simulink model "sampleModel149"  (R2021b)
settings: Solver=VariableStepAuto  StartTime=0.0  StopTime=10.0  RelTol=1e-3
undefined symbols (not defined in the file or in its folder): DiscIntNeverNeededParam, Newton, Raphson
libraries: simulink x9, slpidlib x3
settings Model: Creator=user  LastModifiedBy=user

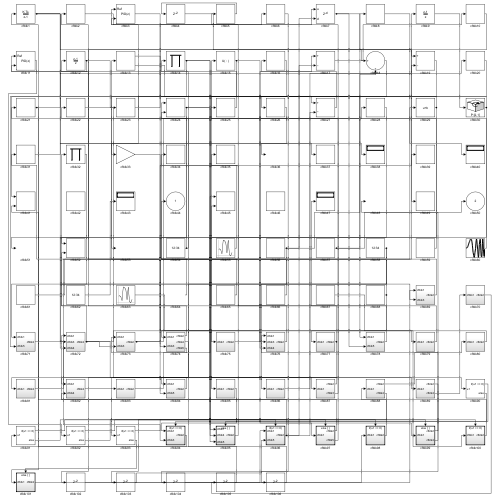
[thumbnail: Simulink's stored preview of the top-level diagram]
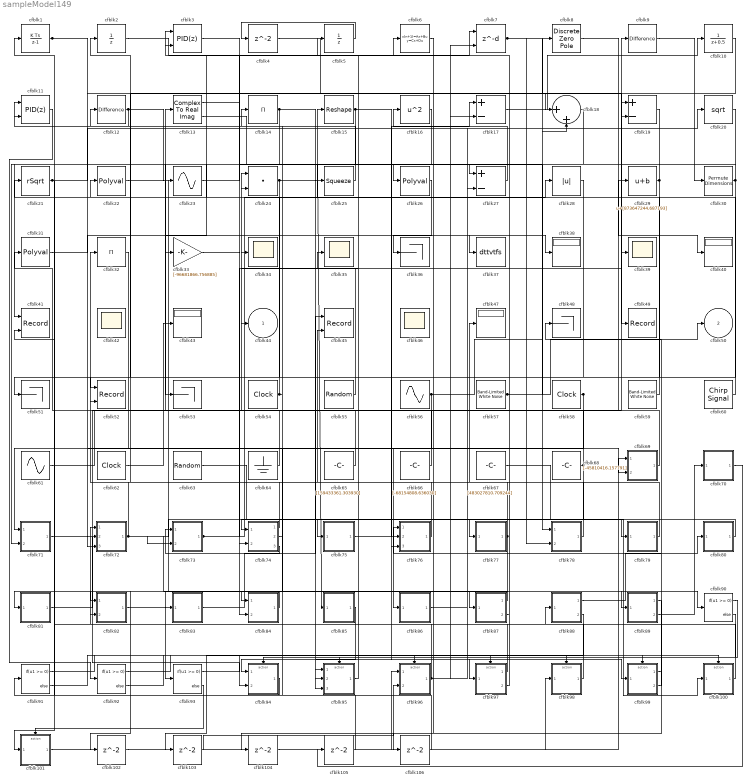
== system sampleModel149 ==
  cfblk1 : DiscreteIntegrator  ICPrevOutput=DiscIntNeverNeededParam  ICPrevScaledInput=DiscIntNeverNeededParam
  cfblk10 : DiscreteTransferFcn  SampleTime=1
  cfblk100 : Subsystem  TreatAsAtomicUnit=on
  cfblk101 : Subsystem  TreatAsAtomicUnit=on
  cfblk{4,102..106} (6 alike) : Delay  SampleTime=1
  cfblk11 : slpidlib/PID Controller (2DOF)  Controller=PID  Form=Parallel  TimeDomain=Discrete-time  UseExternalTs=off  SampleTime=1  IntegratorMethod=Forward Euler  FilterMethod=Forward Euler  ControllerParametersSource=internal  P=1  I=1  D=0  UseFilter=on  N=100  b=1  c=1  TunerSelectOption=Transfer Function Based (PID Tuner App)  InitialConditionSource=internal  InitialConditionForIntegrator=0  InitialConditionForFilter=0  DifferentiatorICPrevScaledInput=0  ExternalReset=none  TrackingMode=off  Kt=1  LimitOutput=off  SatLimitsSource=internal  UpperSaturationLimit=inf  LowerSaturationLimit=-inf  LinearizeAsGain=off  AntiWindupMode=none  Kb=1  POutMin=[]  POutMax=[]  IOutMin=[]  IOutMax=[]  DOutMin=[]  DOutMax=[]  NOutMin=[]  NOutMax=[]  bOutMin=[]  bOutMax=[]  cOutMin=[]  cOutMax=[]  SumOutMin=[]  SumOutMax=[]  SaturationOutMin=[]  SaturationOutMax=[]  PParamMin=[]  PParamMax=[]  IParamMin=[]  IParamMax=[]  DParamMin=[]  DParamMax=[]  NParamMin=[]  NParamMax=[]  bParamMin=[]  bParamMax=[]  cParamMin=[]  cParamMax=[]  KbParamMin=[]  KbParamMax=[]  KtParamMin=[]  KtParamMax=[]  KbOutMin=[]  KbOutMax=[]  KtOutMin=[]  KtOutMax=[]  IntegratorOutMin=[]  IntegratorOutMax=[]  FilterOutMin=[]  FilterOutMax=[]  SumI1OutMin=[]  SumI1OutMax=[]  SumI2OutMin=[]  SumI2OutMax=[]  SumI3OutMin=[]  SumI3OutMax=[]  SumI4OutMin=[]  SumI4OutMax=[]  SumDOutMin=[]  SumDOutMax=[]  Sum1OutMin=[]  Sum1OutMax=[]  Sum2OutMin=[]  Sum2OutMax=[]  Sum3OutMin=[]  Sum3OutMax=[]  DifferentiatorOutMin=[]  DifferentiatorOutMax=[]  FilterDiffOutCoefMin=[]  FilterDiffOutCoefMax=[]  ReciprocalOutMin=[]  ReciprocalOutMax=[]  SumDenOutMin=[]  SumDenOutMax=[]  SumNumOutMin=[]  SumNumOutMax=[]  DivideOutMin=[]  DivideOutMax=[]  UdiffTsProdOutMin=[]  UdiffTsProdOutMax=[]  NTsProdOutMin=[]  NTsProdOutMax=[]  UintegralTsProdOutMin=[]  UintegralTsProdOutMax=[]  UngainTsProdOutMin=[]  UngainTsProdOutMax=[]  IntegratorContinuousStateAttributes=''  IntegratorStateMustResolveToSignalObject=off  IntegratorRTWStateStorageClass=Auto  FilterContinuousStateAttributes=''  FilterStateMustResolveToSignalObject=off  FilterRTWStateStorageClass=Auto  ParallelPVariant=InternalParameters  IdealPVariant=Disabled  IVariant=InternalParameters  DVariant=InternalParameters  bVariant=InternalParameters  cVariant=InternalParameters  IntegratorVariant=Discrete  SatVariant=Disabled  AWVariant=Passthrough  PCopyVariant=Disabled  TRVariant=Disabled  FdbkBlocksVariant=Forward  IdealPFdbkVariant=Disabled  SatFdbkVariant=Disabled  DerivativeFilterVariant=ForwardEulerFilter  NVariant=InternalParameters  NCopyVariant=Disabled  FilterICVariant=InternalICsFilter  IntegratorICVariant=InternalICs  ExternalResetVariant=Disabled  TRSumVariant=Passthrough  SumFdbkVariant=Disabled  SumVariant=Sum_PID  TsampFilterVariant=InternalTs  TsampNgainVariant=Passthrough  TsampIntegralVariant=Passthrough  ExternalSaturationOutDataTypeStr=Inherit: Same as second input
      settings: SourceProductBaseCode=SL
  cfblk12 : simulink/Discrete/Difference  ICPrevInput=0.0  OutMin=[]  OutMax=[]  OutDataTypeStr=Inherit: Inherit via back propagation  OutDataType=fixdt(1, 16)  OutScaling=2^-10  DoSatur=off
  cfblk13 : ComplexToRealImag
  cfblk14 : Product  Inputs=*
  cfblk15 : Reshape
  cfblk16 : Math  Operator=square  SaturateOnIntegerOverflow=on
  cfblk17 : Sum  Inputs=+-
  cfblk18 : Sum  Inputs=|++
  cfblk19 : Sum  Inputs=+-
  cfblk2 : UnitDelay  HasFrameUpgradeWarning=on
  cfblk20 : Sqrt  SaturateOnIntegerOverflow=on
  cfblk21 : Sqrt  Operator=rSqrt  AlgorithmType=Newton-Raphson  SaturateOnIntegerOverflow=on
  cfblk22 : Polyval  Coefs=[ +2.081618890e-019, -1.441693666e-014, +4.719686976e-010, -8.536869453e-006, +1.621573104e-001, -8.087801117e+001 ]
  cfblk23 : Sin  TimeSource=Use external signal  SampleTime=0
  cfblk24 : DotProduct  InputSameDT=on  OutDataTypeStr=Inherit: Inherit via internal rule
  cfblk25 : Squeeze
  cfblk26 : Polyval  Coefs=[ +2.081618890e-019, -1.441693666e-014, +4.719686976e-010, -8.536869453e-006, +1.621573104e-001, -8.087801117e+001 ]
  cfblk27 : Sum  Inputs=+-
  cfblk28 : Abs
  cfblk29 : Bias  Bias=[873647244.687193]
  cfblk3 : slpidlib/PID Controller (2DOF)  Controller=PID  Form=Parallel  TimeDomain=Discrete-time  UseExternalTs=off  SampleTime=1  IntegratorMethod=Forward Euler  FilterMethod=Forward Euler  ControllerParametersSource=internal  P=1  I=1  D=0  UseFilter=on  N=100  b=1  c=1  TunerSelectOption=Transfer Function Based (PID Tuner App)  InitialConditionSource=internal  InitialConditionForIntegrator=0  InitialConditionForFilter=0  DifferentiatorICPrevScaledInput=0  ExternalReset=none  TrackingMode=off  Kt=1  LimitOutput=off  SatLimitsSource=internal  UpperSaturationLimit=inf  LowerSaturationLimit=-inf  LinearizeAsGain=off  AntiWindupMode=none  Kb=1  POutMin=[]  POutMax=[]  IOutMin=[]  IOutMax=[]  DOutMin=[]  DOutMax=[]  NOutMin=[]  NOutMax=[]  bOutMin=[]  bOutMax=[]  cOutMin=[]  cOutMax=[]  SumOutMin=[]  SumOutMax=[]  SaturationOutMin=[]  SaturationOutMax=[]  PParamMin=[]  PParamMax=[]  IParamMin=[]  IParamMax=[]  DParamMin=[]  DParamMax=[]  NParamMin=[]  NParamMax=[]  bParamMin=[]  bParamMax=[]  cParamMin=[]  cParamMax=[]  KbParamMin=[]  KbParamMax=[]  KtParamMin=[]  KtParamMax=[]  KbOutMin=[]  KbOutMax=[]  KtOutMin=[]  KtOutMax=[]  IntegratorOutMin=[]  IntegratorOutMax=[]  FilterOutMin=[]  FilterOutMax=[]  SumI1OutMin=[]  SumI1OutMax=[]  SumI2OutMin=[]  SumI2OutMax=[]  SumI3OutMin=[]  SumI3OutMax=[]  SumI4OutMin=[]  SumI4OutMax=[]  SumDOutMin=[]  SumDOutMax=[]  Sum1OutMin=[]  Sum1OutMax=[]  Sum2OutMin=[]  Sum2OutMax=[]  Sum3OutMin=[]  Sum3OutMax=[]  DifferentiatorOutMin=[]  DifferentiatorOutMax=[]  FilterDiffOutCoefMin=[]  FilterDiffOutCoefMax=[]  ReciprocalOutMin=[]  ReciprocalOutMax=[]  SumDenOutMin=[]  SumDenOutMax=[]  SumNumOutMin=[]  SumNumOutMax=[]  DivideOutMin=[]  DivideOutMax=[]  UdiffTsProdOutMin=[]  UdiffTsProdOutMax=[]  NTsProdOutMin=[]  NTsProdOutMax=[]  UintegralTsProdOutMin=[]  UintegralTsProdOutMax=[]  UngainTsProdOutMin=[]  UngainTsProdOutMax=[]  IntegratorContinuousStateAttributes=''  IntegratorStateMustResolveToSignalObject=off  IntegratorRTWStateStorageClass=Auto  FilterContinuousStateAttributes=''  FilterStateMustResolveToSignalObject=off  FilterRTWStateStorageClass=Auto  ParallelPVariant=InternalParameters  IdealPVariant=Disabled  IVariant=InternalParameters  DVariant=InternalParameters  bVariant=InternalParameters  cVariant=InternalParameters  IntegratorVariant=Discrete  SatVariant=Disabled  AWVariant=Passthrough  PCopyVariant=Disabled  TRVariant=Disabled  FdbkBlocksVariant=Forward  IdealPFdbkVariant=Disabled  SatFdbkVariant=Disabled  DerivativeFilterVariant=ForwardEulerFilter  NVariant=InternalParameters  NCopyVariant=Disabled  FilterICVariant=InternalICsFilter  IntegratorICVariant=InternalICs  ExternalResetVariant=Disabled  TRSumVariant=Passthrough  SumFdbkVariant=Disabled  SumVariant=Sum_PID  TsampFilterVariant=InternalTs  TsampNgainVariant=Passthrough  TsampIntegralVariant=Passthrough  ExternalSaturationOutDataTypeStr=Inherit: Same as second input
      settings: SourceProductBaseCode=SL
  cfblk30 : PermuteDimensions
  cfblk31 : Polyval  Coefs=[ +2.081618890e-019, -1.441693666e-014, +4.719686976e-010, -8.536869453e-006, +1.621573104e-001, -8.087801117e+001 ]
  cfblk32 : Product  Inputs=*
  cfblk33 : Gain  Gain=[-96681866.756885]
  cfblk{34..35,39,42,46} (5 alike) : Scope
      cfblk42 settings: Floating=on
      cfblk46 settings: Floating=on
  cfblk{36,48,51,53} (4 alike) : Terminator
  cfblk37 : ToWorkspace  VariableName=dttvtfs  SaveFormat=Timeseries  SampleTime=-1
  cfblk{38,40,43,47} (4 alike) : Display
  cfblk41 : Record  FileSettingsInternal="{\"entries\":[{\"content\":{\"excelSettings\":{\"content\":{},\"type\":\"Streamout.ExcelSettings\"}},\"type\":\"Streamout.FileSettingStorage\",\"uuid\":\"677ef7f0-aff7-4f23-a399-6c1ba6bb11ad\"}],\"packageUris\":[\"http://schema.mathworks.com/mf0/streamout_blocks/R2020a\"],\"version\":\"1.0\"}"  Layout=[1 1]  SignalsInternal="{\"entries\":[{\"content\":{\"signals\":[{\"content\":{\"blockPath\":[\"sampleModel149/cfblk41\"],\"channel\":[],\"dimensions\":[1],\"domain\":\"sampleModel149/cfblk41\",\"lineColor\":\"#a2142f\",\"plots\":[1],\"port\":1,\"sid\":[\"\"],\"signalID\":5432,\"signalName\":\"cfblk19\"},\"type\":\"RecordBlkView.Signal\",\"uuid\":\"c9c64e99-b97b-4934-8607-4a52140b3292\"},{\"content\":{\"blockPath\":[\"sampleModel149/cfblk41\"],\"channel\":[],\"dimensions\":[1,1],\"domain\":\"sampleModel149/cfblk41\",\"lineColor\":\"#139fff\",\"plots\":[1],\"port\":2,\"sid\":[\"\"],\"signalID\":5436,\"signalName\":\"cfblk98\"},\"type\":\"RecordBlkView.Signal\",\"uuid\":\"e3f4b030-1437-455a-8e97-1c66a963d646\"}]},\"type\":\"RecordBlkView.InputSignals\",\"uuid\":\"ff853e2b-74fa-449a-8b5d-28d87580d79c\"}],\"packageUris\":[\"http://schema.mathworks.com/mf0/streamout_blocks/R2020a\"],\"version\":\"1.0\"}"  VisualizationBindings="{\"xyplotplugin\":{\"info\":[{\"series\":[{\"bindingParametersList\":[{\"parameter\":\"X-Axis\",\"signalID\":5432,\"signalName\":\"cfblk19\"},{\"parameter\":\"Y-Axis\",\"signalID\":5436,\"signalName\":\"cfblk98\"}],\"seriesID\":11011}],\"subplotID\":1}]}}"  CompatibilityTag=XY
  cfblk45 : Record  FileSettingsInternal="{\"entries\":[{\"content\":{\"excelSettings\":{\"content\":{},\"type\":\"Streamout.ExcelSettings\"}},\"type\":\"Streamout.FileSettingStorage\",\"uuid\":\"1409c736-9582-47b9-9387-f52cb0728f9d\"}],\"packageUris\":[\"http://schema.mathworks.com/mf0/streamout_blocks/R2020a\"],\"version\":\"1.0\"}"  Layout=[1 1]  SignalsInternal="{\"entries\":[{\"content\":{\"signals\":[{\"content\":{\"blockPath\":[\"sampleModel149/cfblk45\"],\"channel\":[],\"dimensions\":[1],\"domain\":\"sampleModel149/cfblk45\",\"lineColor\":\"#a2142f\",\"plots\":[1],\"port\":1,\"sid\":[\"\"],\"signalID\":5440,\"signalName\":\"cfblk83\"},\"type\":\"RecordBlkView.Signal\",\"uuid\":\"fdb62399-27ef-4b59-8b56-8b24fd231024\"},{\"content\":{\"blockPath\":[\"sampleModel149/cfblk45\"],\"channel\":[],\"dimensions\":[1],\"domain\":\"sampleModel149/cfblk45\",\"lineColor\":\"#139fff\",\"plots\":[1],\"port\":2,\"sid\":[\"\"],\"signalID\":5444,\"signalName\":\"cfblk78\"},\"type\":\"RecordBlkView.Signal\",\"uuid\":\"29c230be-d527-48a2-af4a-0a38f625c53a\"}]},\"type\":\"RecordBlkView.InputSignals\",\"uuid\":\"a810b71f-787a-4438-9690-a1636733047d\"}],\"packageUris\":[\"http://schema.mathworks.com/mf0/streamout_blocks/R2020a\"],\"version\":\"1.0\"}"  VisualizationBindings="{\"xyplotplugin\":{\"info\":[{\"series\":[{\"bindingParametersList\":[{\"parameter\":\"X-Axis\",\"signalID\":5440,\"signalName\":\"cfblk83\"},{\"parameter\":\"Y-Axis\",\"signalID\":5444,\"signalName\":\"cfblk78\"}],\"seriesID\":23420}],\"subplotID\":1}]}}"  CompatibilityTag=XY
  cfblk49 : Record  FileSettingsInternal="{\"entries\":[{\"content\":{\"excelSettings\":{\"content\":{},\"type\":\"Streamout.ExcelSettings\"}},\"type\":\"Streamout.FileSettingStorage\",\"uuid\":\"623240cd-226e-4570-abce-ef017ed00bb4\"}],\"packageUris\":[\"http://schema.mathworks.com/mf0/streamout_blocks/R2020a\"],\"version\":\"1.0\"}"  SignalsInternal="{\"entries\":[{\"content\":{\"signals\":[{\"content\":{\"blockPath\":[\"sampleModel149/cfblk49\"],\"channel\":[],\"dimensions\":[1,1],\"domain\":\"sampleModel149/cfblk49\",\"lineColor\":\"#b746ff\",\"plots\":[1],\"port\":1,\"sid\":[\"\"],\"signalID\":5448,\"signalName\":\"cfblk4\"},\"type\":\"RecordBlkView.Signal\",\"uuid\":\"dca9496e-cca6-4e71-bce4-3e747afdf648\"}]},\"type\":\"RecordBlkView.InputSignals\",\"uuid\":\"d1a2848c-7443-4a4c-8c65-2b393a3907bc\"}],\"packageUris\":[\"http://schema.mathworks.com/mf0/streamout_blocks/R2020a\"],\"version\":\"1.0\"}"  VisualizationBindings="{\"sparklinesplugin\":{\"info\":[{\"bindingParametersList\":[],\"subplotID\":1}]}}"
  cfblk5 : UnitDelay  HasFrameUpgradeWarning=on
  cfblk52 : Record  FileSettingsInternal="{\"entries\":[{\"content\":{\"excelSettings\":{\"content\":{},\"type\":\"Streamout.ExcelSettings\"}},\"type\":\"Streamout.FileSettingStorage\",\"uuid\":\"783af22f-5e4b-4910-9486-9e25a4d682cd\"}],\"packageUris\":[\"http://schema.mathworks.com/mf0/streamout_blocks/R2020a\"],\"version\":\"1.0\"}"  Layout=[1 1]  SignalsInternal="{\"entries\":[{\"content\":{\"signals\":[{\"content\":{\"blockPath\":[\"sampleModel149/cfblk52\"],\"channel\":[],\"dimensions\":[1],\"domain\":\"sampleModel149/cfblk52\",\"lineColor\":\"#a2142f\",\"plots\":[1],\"port\":1,\"sid\":[\"\"],\"signalID\":5452,\"signalName\":\"cfblk10\"},\"type\":\"RecordBlkView.Signal\",\"uuid\":\"96ba5218-7d5b-45e8-8273-5adbd7f1b230\"},{\"content\":{\"blockPath\":[\"sampleModel149/cfblk52\"],\"channel\":[],\"dimensions\":[1],\"domain\":\"sampleModel149/cfblk52\",\"lineColor\":\"#139fff\",\"plots\":[1],\"port\":2,\"sid\":[\"\"],\"signalID\":5456,\"signalName\":\"cfblk72\"},\"type\":\"RecordBlkView.Signal\",\"uuid\":\"7736bef1-80bc-40a6-a6dc-4b0b7e87cbbb\"}]},\"type\":\"RecordBlkView.InputSignals\",\"uuid\":\"bf4e6791-d3c2-4b19-81ce-781291fa686f\"}],\"packageUris\":[\"http://schema.mathworks.com/mf0/streamout_blocks/R2020a\"],\"version\":\"1.0\"}"  VisualizationBindings="{\"xyplotplugin\":{\"info\":[{\"series\":[{\"bindingParametersList\":[{\"parameter\":\"X-Axis\",\"signalID\":5452,\"signalName\":\"cfblk10\"},{\"parameter\":\"Y-Axis\",\"signalID\":5456,\"signalName\":\"cfblk72\"}],\"seriesID\":36571}],\"subplotID\":1}]}}"  CompatibilityTag=XY
  cfblk54 : DigitalClock
  cfblk55 : RandomNumber  Mean=[12730.939790]  Variance=[38106.151862]  Seed=[917276166.000000]  SampleTime=0.1
  cfblk56 : Sin  Amplitude=[-539187090.809875]  Bias=[865771943.360757]  SampleTime=0
  cfblk57 : simulink/Sources/Band-Limited White Noise  Cov=[5876593269.767416]  Ts=0.1  seed=[5045918873.000000]
  cfblk58 : DigitalClock
  cfblk59 : simulink/Sources/Band-Limited White Noise  Cov=[4025642049.334972]  Ts=0.1  seed=[6678384741.000000]
  cfblk6 : DiscreteStateSpace
  cfblk60 : simulink/Sources/Chirp Signal  f1=[-507852172.117441]  T=[-305736108.698477]  f2=[225463785.672512]
  cfblk61 : Sin  Amplitude=[546175675.773895]  Bias=[-136841052.447450]  SampleTime=0
  cfblk62 : DigitalClock
  cfblk63 : RandomNumber  Mean=[-24942.890571]  Variance=[22742.277888]  Seed=[271279025.000000]  SampleTime=0.1
  cfblk64 : Ground
  cfblk65 : Constant  Value=[159433361.303930]  SampleTime=1
  cfblk66 : Constant  Value=[-68154808.636030]  SampleTime=1
  cfblk67 : Constant  Value=[483027810.709244]  SampleTime=1
  cfblk68 : Constant  Value=[-45810416.157791]  SampleTime=1
  cfblk69 : Subsystem
  cfblk7 : Delay  DelayLengthSource=Input port  SampleTime=1
      settings: InputPortMap=u0,p1
  cfblk70 : Subsystem
  cfblk71 : Subsystem
  cfblk72 : Subsystem
  cfblk73 : Subsystem
  cfblk74 : Subsystem
  cfblk75 : Subsystem
  cfblk76 : Subsystem
  cfblk77 : Subsystem
  cfblk78 : Subsystem
  cfblk79 : Subsystem
  cfblk8 : DiscreteZeroPole  Poles=[0 0.5]  Gain=1
  cfblk80 : Subsystem
  cfblk81 : Subsystem
  cfblk82 : Subsystem
  cfblk83 : Subsystem
  cfblk84 : Subsystem
  cfblk85 : Subsystem
  cfblk86 : Subsystem
  cfblk87 : Subsystem
  cfblk88 : Subsystem
  cfblk89 : Subsystem
  cfblk9 : simulink/Discrete/Difference  ICPrevInput=0.0  OutMin=[]  OutMax=[]  OutDataTypeStr=Inherit: Inherit via back propagation  OutDataType=fixdt(1, 16)  OutScaling=2^-10  DoSatur=off
  cfblk{90..93} (4 alike) : If  IfExpression=u1 >= 0  SampleTime=1
  cfblk94 : Subsystem  TreatAsAtomicUnit=on
  cfblk95 : Subsystem  TreatAsAtomicUnit=on
  cfblk96 : Subsystem  TreatAsAtomicUnit=on
  cfblk97 : Subsystem  TreatAsAtomicUnit=on
  cfblk98 : Subsystem  TreatAsAtomicUnit=on
  cfblk99 : Subsystem  TreatAsAtomicUnit=on
  cfblk44 : Outport
  cfblk50 : Outport  Port=2
  wires:
  cfblk17/1 -> cfblk10/1
  cfblk74/1(cfblk2) -> cfblk32/1
  cfblk19/1 -> cfblk41/1
  cfblk27/1 -> cfblk16/1
  cfblk69/1(cfblk2) -> cfblk24/1
  cfblk11/1 -> cfblk92/1
  cfblk99/1(cfblk2) -> cfblk48/1
  cfblk76/1(cfblk2) -> cfblk2/1
  cfblk10/1 -> cfblk52/1
  cfblk15/1 -> cfblk97/1(cfblk1), cfblk95/3(cfblk5)
  cfblk84/1(cfblk2) -> cfblk81/1(cfblk1)
  cfblk81/1(cfblk2) -> cfblk9/1
  cfblk8/1 -> cfblk40/1
  cfblk54/1 -> cfblk14/1, cfblk3/2
  cfblk28/1 -> cfblk101/1(cfblk1)
  cfblk26/1 -> cfblk36/1
  cfblk60/1 -> cfblk15/1
  cfblk67/1 -> cfblk100/1(cfblk1)
  cfblk24/1 -> cfblk85/1(cfblk1), cfblk99/1(cfblk1), cfblk84/2(cfblk5)
  cfblk66/1 -> cfblk13/1
  cfblk2/1 -> cfblk6/1
  cfblk73/1(cfblk2) -> cfblk28/1, cfblk39/1
  cfblk72/1(cfblk2) -> cfblk75/1(cfblk1), cfblk73/2(cfblk3), cfblk89/1(cfblk1), cfblk52/2
  cfblk22/1 -> cfblk90/1
  cfblk59/1 -> cfblk22/1
  cfblk14/1 -> cfblk79/1(cfblk1), cfblk87/1(cfblk1), cfblk71/2(cfblk5)
  cfblk68/1 -> cfblk74/1(cfblk1), cfblk44/1
  cfblk30/1 -> cfblk25/1, cfblk95/2(cfblk4)
  cfblk56/1 -> cfblk86/1(cfblk1), cfblk18/2, cfblk7/2
  cfblk65/1 -> cfblk31/1
  cfblk18/1 -> cfblk53/1
  cfblk99/2(cfblk4) -> cfblk76/1(cfblk1)
  cfblk94/1(cfblk2) -> cfblk91/1
  cfblk21/1 -> cfblk20/1, cfblk51/1
  cfblk57/1 -> cfblk8/1, cfblk50/1
  cfblk88/1(cfblk2) -> cfblk80/1(cfblk1)
  cfblk63/1 -> cfblk95/1(cfblk1)
  cfblk25/1 -> cfblk11/1
  cfblk5/1 -> cfblk4/1
  cfblk1/1 -> cfblk37/1, cfblk18/1, cfblk69/2(cfblk3)
  cfblk75/1(cfblk2) -> cfblk17/1
  cfblk80/1(cfblk2) -> cfblk77/1(cfblk1)
  cfblk83/1(cfblk2) -> cfblk45/1
  cfblk62/1 -> cfblk43/1
  cfblk85/1(cfblk2) -> cfblk94/1(cfblk1)
  cfblk4/1 -> cfblk49/1
  cfblk55/1 -> cfblk34/1
  cfblk61/1 -> cfblk29/1
  cfblk12/1 -> cfblk23/1, cfblk11/2
  cfblk98/1(cfblk2) -> cfblk41/2
  cfblk58/1 -> cfblk84/1(cfblk1), cfblk72/3(cfblk4)
  cfblk3/1 -> cfblk27/1
  cfblk82/1(cfblk2) -> cfblk93/1
  cfblk13/1 -> cfblk74/2(cfblk3)
  cfblk13/2 -> cfblk78/1(cfblk1)
  cfblk9/1 -> cfblk30/1
  cfblk95/1(cfblk2) -> cfblk35/1
  cfblk87/1(cfblk2) -> cfblk83/1(cfblk1)
  cfblk97/1(cfblk2) -> cfblk72/1(cfblk1)
  cfblk64/1 -> cfblk12/1
  cfblk33/1 -> cfblk76/2(cfblk3)
  cfblk20/1 -> cfblk76/3(cfblk4)
  cfblk101/1(cfblk2) -> cfblk98/1(cfblk1)
  cfblk32/1 -> cfblk71/1(cfblk1)
  cfblk86/1(cfblk2) -> cfblk27/2
  cfblk71/1(cfblk2) -> cfblk94/2(cfblk3)
  cfblk78/1(cfblk2) -> cfblk45/2
  cfblk29/1 -> cfblk72/2(cfblk3), cfblk26/1
  cfblk31/1 -> cfblk38/1
  cfblk74/2(cfblk4) -> cfblk82/1(cfblk1)
  cfblk96/1(cfblk2) -> cfblk82/2(cfblk4), cfblk19/2, cfblk17/2
  cfblk23/1 -> cfblk7/1
  cfblk97/2(cfblk5) -> cfblk21/1
  cfblk7/1 -> cfblk19/1, cfblk78/2(cfblk5)
  cfblk74/3(cfblk5) -> cfblk73/1(cfblk1)
  cfblk100/1(cfblk2) -> cfblk88/1(cfblk1)
  cfblk77/1(cfblk2) -> cfblk47/1, cfblk102/1
  cfblk79/1(cfblk2) -> cfblk5/1
  cfblk16/1 -> cfblk33/1
  cfblk89/2(cfblk4) -> cfblk70/1(cfblk1)
  cfblk87/2(cfblk3) -> cfblk3/1
  cfblk90/1 -> cfblk94/Action
  cfblk90/2 -> cfblk95/Action
  cfblk91/1 -> cfblk96/Action
  cfblk91/2 -> cfblk97/Action
  cfblk92/1 -> cfblk98/Action
  cfblk92/2 -> cfblk99/Action
  cfblk93/1 -> cfblk100/Action
  cfblk93/2 -> cfblk101/Action
  cfblk102/1 -> cfblk69/1(cfblk1)
  cfblk88/2(cfblk4) -> cfblk103/1
  cfblk103/1 -> cfblk96/2(cfblk5)
  cfblk89/1(cfblk2) -> cfblk104/1
  cfblk104/1 -> cfblk96/1(cfblk1)
  cfblk70/1(cfblk2) -> cfblk105/1
  cfblk105/1 -> cfblk24/2
  cfblk6/1 -> cfblk106/1
  cfblk106/1 -> cfblk1/1

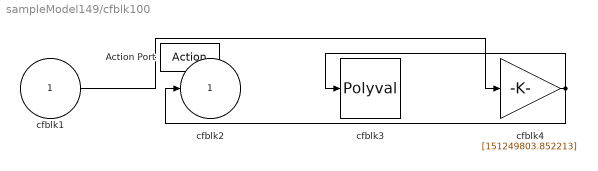
== system sampleModel149/cfblk100 ==
  cfblk1 : Inport
  Action Port : ActionPort  ActionPortLabel=if(u1 >= 0)
  cfblk3 : Polyval  Coefs=[ +2.081618890e-019, -1.441693666e-014, +4.719686976e-010, -8.536869453e-006, +1.621573104e-001, -8.087801117e+001 ]
  cfblk4 : Gain  Gain=[151249803.852213]
  cfblk2 : Outport
  wires:
  cfblk4/1 -> cfblk2/1, cfblk3/1
  cfblk1/1 -> cfblk4/1

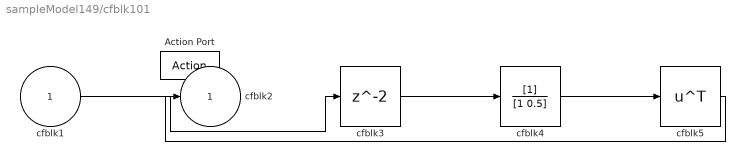
== system sampleModel149/cfblk101 ==
  cfblk1 : Inport
  Action Port : ActionPort  ActionPortLabel=else
  cfblk3 : Delay
  cfblk4 : DiscreteFilter
  cfblk5 : Math  Operator=transpose  SaturateOnIntegerOverflow=on
  cfblk2 : Outport
  wires:
  cfblk1/1 -> cfblk3/1
  cfblk3/1 -> cfblk4/1
  cfblk4/1 -> cfblk5/1
  cfblk5/1 -> cfblk2/1

== system sampleModel149/cfblk69 ==
  cfblk1 : Inport
  cfblk3 : Inport  Port=2
  cfblk2 : Outport
  wires:
  cfblk3/1 -> cfblk2/1

== system sampleModel149/cfblk70 ==
  cfblk1 : Inport
  cfblk3 : Assignment  DiagnosticForDimensions=Warning  IndexOptions=Index vector (dialog)  Indices=1  OutputSizes=1
  cfblk4 : Constant  Value=[-242682656.230599]  SampleTime=1
  cfblk2 : Outport
  wires:
  cfblk4/1 -> cfblk3/1
  cfblk1/1 -> cfblk2/1, cfblk3/2

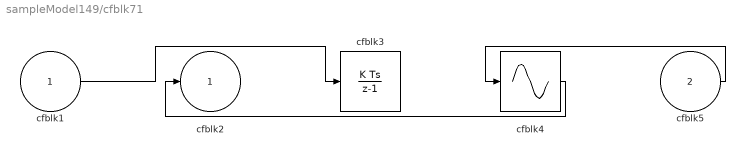
== system sampleModel149/cfblk71 ==
  cfblk1 : Inport
  cfblk5 : Inport  Port=2
  cfblk3 : DiscreteIntegrator  ICPrevOutput=DiscIntNeverNeededParam  ICPrevScaledInput=DiscIntNeverNeededParam
  cfblk4 : Sin  TimeSource=Use external signal  SampleTime=0
  cfblk2 : Outport
  wires:
  cfblk5/1 -> cfblk4/1
  cfblk4/1 -> cfblk2/1
  cfblk1/1 -> cfblk3/1

== system sampleModel149/cfblk72 ==
  cfblk1 : Inport
  cfblk3 : Inport  Port=2
  cfblk4 : Inport  Port=3
  cfblk2 : Outport
  wires:
  cfblk3/1 -> cfblk2/1

== system sampleModel149/cfblk73 ==
  cfblk1 : Inport
  cfblk3 : Inport  Port=2
  cfblk2 : Outport
  wires:
  cfblk1/1 -> cfblk2/1

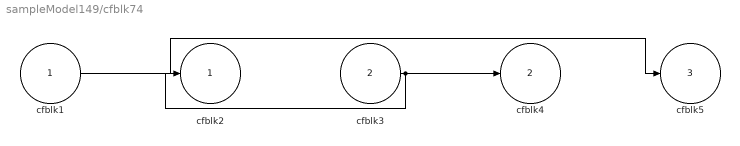
== system sampleModel149/cfblk74 ==
  cfblk1 : Inport
  cfblk3 : Inport  Port=2
  cfblk2 : Outport
  cfblk4 : Outport  Port=2
  cfblk5 : Outport  Port=3
  wires:
  cfblk1/1 -> cfblk5/1
  cfblk3/1 -> cfblk2/1, cfblk4/1

== system sampleModel149/cfblk75 ==
  cfblk1 : Inport
  cfblk3 : Delay  SampleTime=1
  cfblk2 : Outport
  wires:
  cfblk3/1 -> cfblk2/1
  cfblk1/1 -> cfblk3/1

== system sampleModel149/cfblk76 ==
  cfblk1 : Inport
  cfblk3 : Inport  Port=2
  cfblk4 : Inport  Port=3
  cfblk2 : Outport
  wires:
  cfblk3/1 -> cfblk2/1

== system sampleModel149/cfblk77 ==
  cfblk1 : Inport
  cfblk3 : DiscreteTransferFcn  SampleTime=1
  cfblk4 : DiscreteFilter  SampleTime=1
  cfblk2 : Outport
  wires:
  cfblk1/1 -> cfblk3/1
  cfblk4/1 -> cfblk2/1
  cfblk3/1 -> cfblk4/1

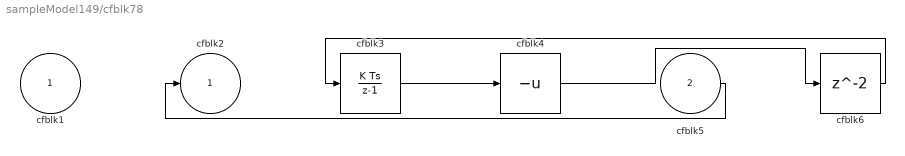
== system sampleModel149/cfblk78 ==
  cfblk1 : Inport
  cfblk5 : Inport  Port=2
  cfblk3 : DiscreteIntegrator  ICPrevOutput=DiscIntNeverNeededParam  ICPrevScaledInput=DiscIntNeverNeededParam
  cfblk4 : UnaryMinus
  cfblk6 : Delay  SampleTime=1
  cfblk2 : Outport
  wires:
  cfblk3/1 -> cfblk4/1
  cfblk5/1 -> cfblk2/1
  cfblk4/1 -> cfblk6/1
  cfblk6/1 -> cfblk3/1

== system sampleModel149/cfblk79 ==
  cfblk1 : Inport
  cfblk3 : Sqrt  SaturateOnIntegerOverflow=on
  cfblk4 : PermuteDimensions
  cfblk2 : Outport
  wires:
  cfblk4/1 -> cfblk3/1
  cfblk3/1 -> cfblk2/1
  cfblk1/1 -> cfblk4/1

== system sampleModel149/cfblk80 ==
  cfblk1 : Inport
  cfblk3 : Delay  DelayLengthSource=Input port  SampleTime=1
      settings: InputPortMap=u0,p1
  cfblk4 : Sum  Inputs=|++
  cfblk2 : Outport
  wires:
  cfblk4/1 -> cfblk3/1
  cfblk1/1 -> cfblk4/1, cfblk3/2, cfblk4/2
  cfblk3/1 -> cfblk2/1

== system sampleModel149/cfblk81 ==
  cfblk1 : Inport
  cfblk3 : simulink/Math Operations/Slider Gain  gain=1  low=0  high=2
  cfblk2 : Outport
  wires:
  cfblk1/1 -> cfblk3/1
  cfblk3/1 -> cfblk2/1

== system sampleModel149/cfblk82 ==
  cfblk1 : Inport
  cfblk4 : Inport  Port=2
  cfblk3 : slpidlib/PID Controller (2DOF)  Controller=PID  Form=Parallel  TimeDomain=Discrete-time  UseExternalTs=off  SampleTime=1  IntegratorMethod=Forward Euler  FilterMethod=Forward Euler  ControllerParametersSource=internal  P=1  I=1  D=0  UseFilter=on  N=100  b=1  c=1  TunerSelectOption=Transfer Function Based (PID Tuner App)  InitialConditionSource=internal  InitialConditionForIntegrator=0  InitialConditionForFilter=0  DifferentiatorICPrevScaledInput=0  ExternalReset=none  TrackingMode=off  Kt=1  LimitOutput=off  SatLimitsSource=internal  UpperSaturationLimit=inf  LowerSaturationLimit=-inf  LinearizeAsGain=off  AntiWindupMode=none  Kb=1  POutMin=[]  POutMax=[]  IOutMin=[]  IOutMax=[]  DOutMin=[]  DOutMax=[]  NOutMin=[]  NOutMax=[]  bOutMin=[]  bOutMax=[]  cOutMin=[]  cOutMax=[]  SumOutMin=[]  SumOutMax=[]  SaturationOutMin=[]  SaturationOutMax=[]  PParamMin=[]  PParamMax=[]  IParamMin=[]  IParamMax=[]  DParamMin=[]  DParamMax=[]  NParamMin=[]  NParamMax=[]  bParamMin=[]  bParamMax=[]  cParamMin=[]  cParamMax=[]  KbParamMin=[]  KbParamMax=[]  KtParamMin=[]  KtParamMax=[]  KbOutMin=[]  KbOutMax=[]  KtOutMin=[]  KtOutMax=[]  IntegratorOutMin=[]  IntegratorOutMax=[]  FilterOutMin=[]  FilterOutMax=[]  SumI1OutMin=[]  SumI1OutMax=[]  SumI2OutMin=[]  SumI2OutMax=[]  SumI3OutMin=[]  SumI3OutMax=[]  SumI4OutMin=[]  SumI4OutMax=[]  SumDOutMin=[]  SumDOutMax=[]  Sum1OutMin=[]  Sum1OutMax=[]  Sum2OutMin=[]  Sum2OutMax=[]  Sum3OutMin=[]  Sum3OutMax=[]  DifferentiatorOutMin=[]  DifferentiatorOutMax=[]  FilterDiffOutCoefMin=[]  FilterDiffOutCoefMax=[]  ReciprocalOutMin=[]  ReciprocalOutMax=[]  SumDenOutMin=[]  SumDenOutMax=[]  SumNumOutMin=[]  SumNumOutMax=[]  DivideOutMin=[]  DivideOutMax=[]  UdiffTsProdOutMin=[]  UdiffTsProdOutMax=[]  NTsProdOutMin=[]  NTsProdOutMax=[]  UintegralTsProdOutMin=[]  UintegralTsProdOutMax=[]  UngainTsProdOutMin=[]  UngainTsProdOutMax=[]  IntegratorContinuousStateAttributes=''  IntegratorStateMustResolveToSignalObject=off  IntegratorRTWStateStorageClass=Auto  FilterContinuousStateAttributes=''  FilterStateMustResolveToSignalObject=off  FilterRTWStateStorageClass=Auto  ParallelPVariant=InternalParameters  IdealPVariant=Disabled  IVariant=InternalParameters  DVariant=InternalParameters  bVariant=InternalParameters  cVariant=InternalParameters  IntegratorVariant=Discrete  SatVariant=Disabled  AWVariant=Passthrough  PCopyVariant=Disabled  TRVariant=Disabled  FdbkBlocksVariant=Forward  IdealPFdbkVariant=Disabled  SatFdbkVariant=Disabled  DerivativeFilterVariant=ForwardEulerFilter  NVariant=InternalParameters  NCopyVariant=Disabled  FilterICVariant=InternalICsFilter  IntegratorICVariant=InternalICs  ExternalResetVariant=Disabled  TRSumVariant=Passthrough  SumFdbkVariant=Disabled  SumVariant=Sum_PID  TsampFilterVariant=InternalTs  TsampNgainVariant=Passthrough  TsampIntegralVariant=Passthrough  ExternalSaturationOutDataTypeStr=Inherit: Same as second input
      settings: SourceProductBaseCode=SL
  cfblk2 : Outport
  wires:
  cfblk1/1 -> cfblk3/1
  cfblk3/1 -> cfblk2/1
  cfblk4/1 -> cfblk3/2

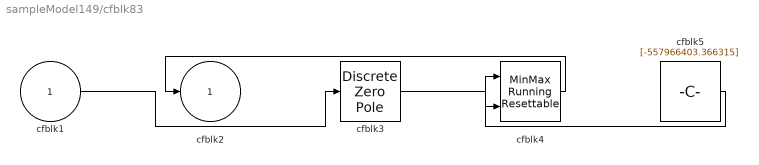
== system sampleModel149/cfblk83 ==
  cfblk1 : Inport
  cfblk3 : DiscreteZeroPole  Poles=[0 0.5]  Gain=1
  cfblk4 : simulink/Math Operations/MinMax Running Resettable  Function=min  vinit=0.0
  cfblk5 : Constant  Value=[-557966403.366315]  SampleTime=1
  cfblk2 : Outport
  wires:
  cfblk4/1 -> cfblk2/1
  cfblk1/1 -> cfblk3/1
  cfblk5/1 -> cfblk4/1
  cfblk3/1 -> cfblk4/2

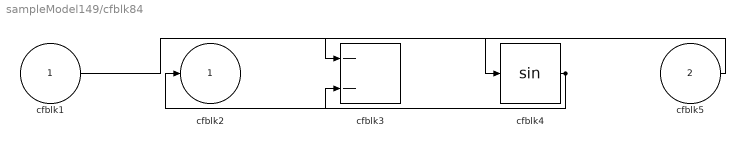
== system sampleModel149/cfblk84 ==
  cfblk1 : Inport
  cfblk5 : Inport  Port=2
  cfblk3 : Sum  Inputs=--
  cfblk4 : Trigonometry
  cfblk2 : Outport
  wires:
  cfblk5/1 -> cfblk3/1
  cfblk4/1 -> cfblk2/1, cfblk3/2
  cfblk1/1 -> cfblk4/1

== system sampleModel149/cfblk85 ==
  cfblk1 : Inport
  cfblk3 : DiscreteFir  SampleTime=1
  cfblk2 : Outport
  wires:
  cfblk3/1 -> cfblk2/1
  cfblk1/1 -> cfblk3/1

== system sampleModel149/cfblk86 ==
  cfblk1 : Inport
  cfblk3 : DiscreteFir  SampleTime=1
  cfblk2 : Outport
  wires:
  cfblk1/1 -> cfblk2/1, cfblk3/1

== system sampleModel149/cfblk87 ==
  cfblk1 : Inport
  cfblk2 : Outport
  cfblk3 : Outport  Port=2
  wires:
  cfblk1/1 -> cfblk2/1, cfblk3/1

== system sampleModel149/cfblk88 ==
  cfblk1 : Inport
  cfblk3 : Rounding
  cfblk2 : Outport
  cfblk4 : Outport  Port=2
  wires:
  cfblk1/1 -> cfblk3/1, cfblk4/1
  cfblk3/1 -> cfblk2/1

== system sampleModel149/cfblk89 ==
  cfblk1 : Inport
  cfblk3 : Bias  Bias=[-688995450.295164]
  cfblk2 : Outport
  cfblk4 : Outport  Port=2
  wires:
  cfblk3/1 -> cfblk2/1
  cfblk1/1 -> cfblk4/1, cfblk3/1

== system sampleModel149/cfblk94 ==
  cfblk1 : Inport
  cfblk3 : Inport  Port=2
  Action Port : ActionPort  ActionPortLabel=if(u1 >= 0)
  cfblk2 : Outport
  wires:
  cfblk1/1 -> cfblk2/1

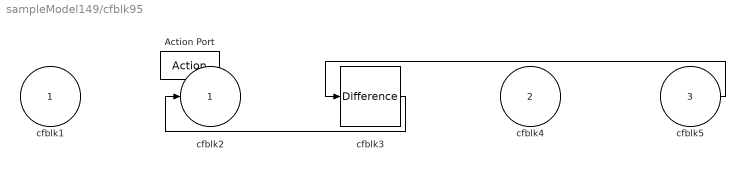
== system sampleModel149/cfblk95 ==
  cfblk1 : Inport
  cfblk4 : Inport  Port=2
  cfblk5 : Inport  Port=3
  Action Port : ActionPort  ActionPortLabel=else
  cfblk3 : simulink/Discrete/Difference  ICPrevInput=0.0  OutMin=[]  OutMax=[]  OutDataTypeStr=Inherit: Inherit via back propagation  OutDataType=fixdt(1, 16)  OutScaling=2^-10  DoSatur=off
  cfblk2 : Outport
  wires:
  cfblk5/1 -> cfblk3/1
  cfblk3/1 -> cfblk2/1

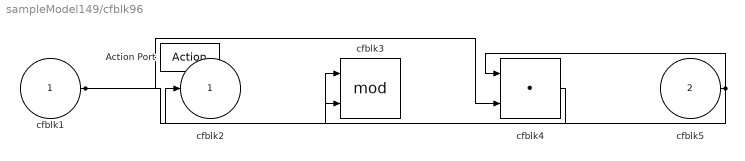
== system sampleModel149/cfblk96 ==
  cfblk1 : Inport
  cfblk5 : Inport  Port=2
  Action Port : ActionPort  ActionPortLabel=if(u1 >= 0)
  cfblk3 : Math  Operator=mod  SaturateOnIntegerOverflow=on
  cfblk4 : DotProduct  InputSameDT=on  OutDataTypeStr=Inherit: Inherit via internal rule
  cfblk2 : Outport
  wires:
  cfblk4/1 -> cfblk2/1
  cfblk5/1 -> cfblk4/1, cfblk3/2
  cfblk1/1 -> cfblk4/2, cfblk3/1

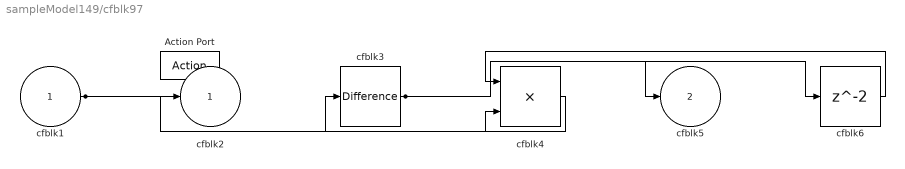
== system sampleModel149/cfblk97 ==
  cfblk1 : Inport
  Action Port : ActionPort  ActionPortLabel=else
  cfblk3 : simulink/Discrete/Difference  ICPrevInput=0.0  OutMin=[]  OutMax=[]  OutDataTypeStr=Inherit: Inherit via back propagation  OutDataType=fixdt(1, 16)  OutScaling=2^-10  DoSatur=off
  cfblk4 : Product
  cfblk6 : Delay
  cfblk2 : Outport
  cfblk5 : Outport  Port=2
  wires:
  cfblk1/1 -> cfblk2/1, cfblk4/2
  cfblk3/1 -> cfblk5/1, cfblk6/1
  cfblk4/1 -> cfblk3/1
  cfblk6/1 -> cfblk4/1

== system sampleModel149/cfblk98 ==
  cfblk1 : Inport
  Action Port : ActionPort  ActionPortLabel=if(u1 >= 0)
  cfblk3 : MinMax  Function=max
  cfblk2 : Outport
  wires:
  cfblk1/1 -> cfblk3/1
  cfblk3/1 -> cfblk2/1

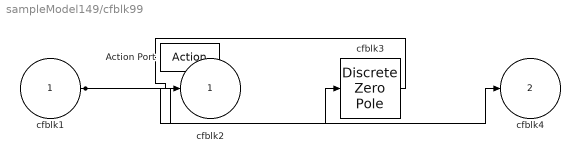
== system sampleModel149/cfblk99 ==
  cfblk1 : Inport
  Action Port : ActionPort  ActionPortLabel=else
  cfblk3 : DiscreteZeroPole  Poles=[0 0.5]  Gain=1  SampleTime=-1
  cfblk2 : Outport
  cfblk4 : Outport  Port=2
  wires:
  cfblk1/1 -> cfblk4/1, cfblk3/1
  cfblk3/1 -> cfblk2/1
